simulink model "stm32_linker"  (R2025a)
settings: Solver=FixedStepAuto  StartTime=0.0  StopTime=inf  FixedStep=0.001  RelTol=1e-3
libraries: dspvision x3, instrumentseriallib x2, dspsnks4 x1, stmutilitieslib x1
settings Model: Creator=User  LastModifiedBy=User

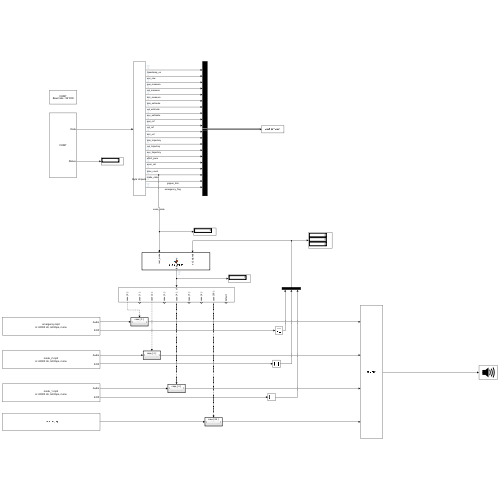
[thumbnail: Simulink's stored preview of the top-level diagram]
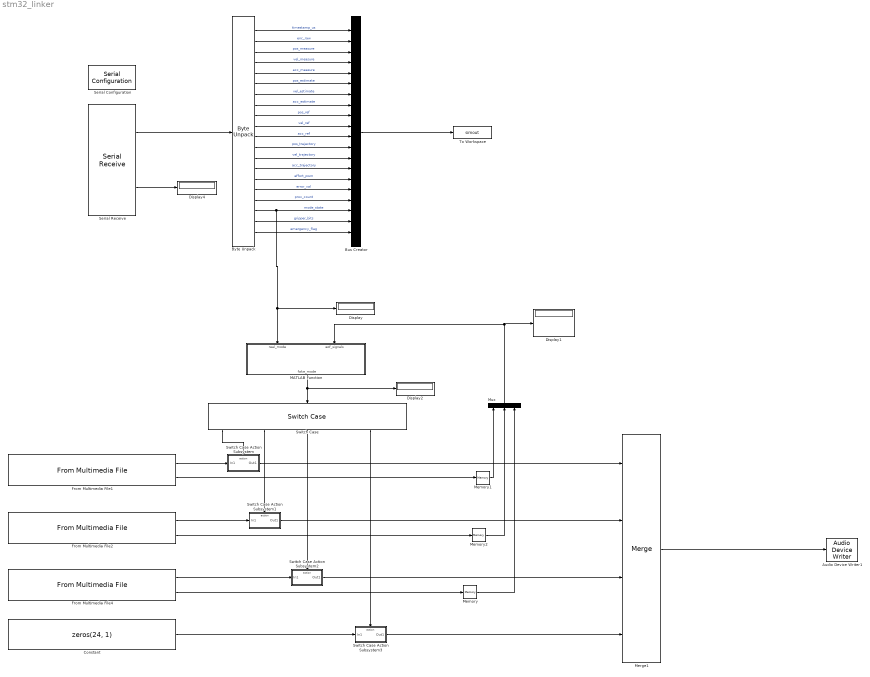
== system stm32_linker ==
  Audio Device Writer1 : dspsnks4/Audio Device Writer  Driver=DirectSound  Device=Headphones (Xiaomi Sound Party)  InheritSampleRate=on  SampleRate=44100  BitDepth=16-bit integer  BufferSize=4096  NumBuffers=10  DefaultOutputChannelMapping=on  OutputChannelMapping=1:2  OutputNumUnderrunSamples=off  DriverIdx=1  DeviceWarnFlag=''
  Bus Creator : BusCreator  Inputs=20
  Byte Unpack : stmutilitieslib/Byte Unpack  dimensions={1, 1, 1, 1, 1, 1, 1, 1, 1, 1, 1, 1, 1, 1, 1, 1, 1,1,1,1}  datatypes={'uint32', 'int32', 'single', 'single', 'single', 'single', 'single', 'single', 'single', 'single', 'single', 'single', 'single', 'single', 'single', 'single', 'int16', 'uint16', 'uint8', 'uint8'}  byteAlign=1  blockPlatform=stm32f4discovery
  Constant : Constant  Value=zeros(24, 1)
  Display{,1..2,4} (4 alike) : Display
  From Multimedia File1 : dspvision/From Multimedia File  inputFilename=C:\Users\User\Documents\GitHub\studioG4_system_modelling\MATLAB_DEBUGGER\mp3\emergency.mp3  readRange=[1 Inf]  loop=on  numPlays=inf  outputStreams=Audio only  videoDataType=single  audioDataType=double  inheritSampleTime=off  userDefinedSampleTime=0.001  noAudioOutput=off  isIntensityVideo=off  fourcc=RGB  colorVideoFormat=Separate color signals  outputEOF=on  dataOrg=Column-major  audioFrameSize=24  computeAudioFrameSize=off  outSamplingMode=Sample based
      settings: LibrarySourceBlock=audiosources/From Multimedia File
  From Multimedia File2 : dspvision/From Multimedia File  inputFilename=C:\Users\User\Documents\GitHub\studioG4_system_modelling\MATLAB_DEBUGGER\mp3\mode_2.mp3  readRange=[1 Inf]  loop=on  numPlays=inf  outputStreams=Audio only  videoDataType=single  audioDataType=double  inheritSampleTime=off  userDefinedSampleTime=0.001  noAudioOutput=off  isIntensityVideo=off  fourcc=RGB  colorVideoFormat=Separate color signals  outputEOF=on  dataOrg=Column-major  audioFrameSize=24  computeAudioFrameSize=off  outSamplingMode=Sample based
      settings: LibrarySourceBlock=audiosources/From Multimedia File
  From Multimedia File4 : dspvision/From Multimedia File  inputFilename=C:\Users\User\Documents\GitHub\studioG4_system_modelling\MATLAB_DEBUGGER\mp3\mode_1.mp3  readRange=[1 Inf]  loop=on  numPlays=inf  outputStreams=Audio only  videoDataType=single  audioDataType=double  inheritSampleTime=off  userDefinedSampleTime=0.001  noAudioOutput=off  isIntensityVideo=off  fourcc=RGB  colorVideoFormat=Separate color signals  outputEOF=on  dataOrg=Column-major  audioFrameSize=24  computeAudioFrameSize=off  outSamplingMode=Sample based
      settings: LibrarySourceBlock=audiosources/From Multimedia File
  MATLAB Function : MATLAB Function  TreatAsAtomicUnit=on
  Memory : Memory
  Memory1 : Memory
  Memory2 : Memory
  Merge1 : Merge  Inputs=4
  Mux : Mux  Inputs=3
  Serial Configuration : instrumentseriallib/Serial Configuration  Priority=-200000  PortSel=COM7  Port=COM7  ComPort=COM7  BaudRate=921000  DataBits=8  Parity=none  StopBits=1  ByteOrder=little-endian  FlowControl=none  Timeout=10  SimulateUsing=Interpreted execution  BlockInModel=on  aMode=1
      settings: LibrarySourceBlock=embeddedtargetslib/Host Communication/Serial Configuration
  Serial Receive : instrumentseriallib/Serial Receive  Priority=1  PortSel=COM7  Port=COM7  ComPort=COM7  DataType=uint8  SaveDataType=uint8  ToggleHeader=on  Header=[170 170 170 170]  ToggleDataSize=on  DataSize=[70 1]  ToggleTerminator=off  Terminator=Custom terminator  CustomTerminator=[]  InputFormat=Column major  EnableBlockingMode=off  ActionDataUnavailable=Output last received value  ActionWhenDataUnavailable=Output last received value  CustomValue=0  SampleTime=0.001  SimulateUsing=Interpreted execution  BlockInModel=on  aMode=1  LibraryInUse=instrumentlib
      settings: LibrarySourceBlock=embeddedtargetslib/Host Communication/Serial Receive
  Switch Case : SwitchCase  CaseConditions={0,1,2,3,4,5,6,99}
  Switch Case Action Subsystem : Subsystem  TreatAsAtomicUnit=on
  Switch Case Action Subsystem1 : Subsystem  TreatAsAtomicUnit=on
  Switch Case Action Subsystem2 : Subsystem  TreatAsAtomicUnit=on
  Switch Case Action Subsystem3 : Subsystem  TreatAsAtomicUnit=on
  To Workspace : ToWorkspace  VariableName=simout  SaveFormat=Timeseries  SampleTime=-1
  wires:
  Bus Creator/1 -> To Workspace/1
  Serial Receive/1 -> Byte Unpack/1
  Serial Receive/2 -> Display4/1
  Byte Unpack/1 -> Bus Creator/1  "timestamp_us"
  Byte Unpack/2 -> Bus Creator/2  "enc_raw"
  Byte Unpack/3 -> Bus Creator/3  "pos_measure"
  Byte Unpack/4 -> Bus Creator/4  "vel_measure"
  Byte Unpack/5 -> Bus Creator/5  "acc_measure"
  Byte Unpack/6 -> Bus Creator/6  "pos_estimate"
  Byte Unpack/7 -> Bus Creator/7  "vel_estimate"
  Byte Unpack/8 -> Bus Creator/8  "acc_estimate"
  Byte Unpack/9 -> Bus Creator/9  "pos_ref"
  Byte Unpack/10 -> Bus Creator/10  "vel_ref"
  Byte Unpack/11 -> Bus Creator/11  "acc_ref"
  Byte Unpack/12 -> Bus Creator/12  "pos_trajectory"
  Byte Unpack/13 -> Bus Creator/13  "vel_trajectory"
  Byte Unpack/14 -> Bus Creator/14  "acc_trajectory"
  Byte Unpack/15 -> Bus Creator/15  "effort_pwm"
  Byte Unpack/16 -> Bus Creator/16  "error_val"
  Byte Unpack/17 -> Bus Creator/17  "prox_count"
  Byte Unpack/18 -> Bus Creator/18, Display/1, MATLAB Function/1(real_mode)  "mode_state"
  Byte Unpack/19 -> Bus Creator/19  "gripper_bits"
  Byte Unpack/20 -> Bus Creator/20  "emergency_flag"
  Merge1/1 -> Audio Device Writer1/1
  From Multimedia File1/1 -> Switch Case Action Subsystem/1(In1)
  From Multimedia File2/1 -> Switch Case Action Subsystem1/1(In1)
  From Multimedia File4/1 -> Switch Case Action Subsystem2/1(In1)
  Switch Case Action Subsystem2/1(Out1) -> Merge1/3
  Switch Case Action Subsystem1/1(Out1) -> Merge1/2
  Switch Case Action Subsystem/1(Out1) -> Merge1/1
  Switch Case/3 -> Switch Case Action Subsystem1/Action
  From Multimedia File4/2 -> Memory/1
  From Multimedia File2/2 -> Memory2/1
  From Multimedia File1/2 -> Memory1/1
  Memory1/1 -> Mux/1
  Memory2/1 -> Mux/2
  Memory/1 -> Mux/3
  Mux/1 -> MATLAB Function/2(eof_signals), Display1/1
  MATLAB Function/1(fake_mode) -> Display2/1, Switch Case/1
  Switch Case/5 -> Switch Case Action Subsystem2/Action
  Switch Case/8 -> Switch Case Action Subsystem3/Action
  Switch Case Action Subsystem3/1(Out1) -> Merge1/4
  Constant/1 -> Switch Case Action Subsystem3/1(In1)
  Switch Case/1 -> Switch Case Action Subsystem/Action

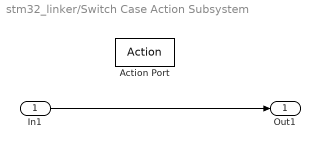
== system stm32_linker/Switch Case Action Subsystem ==
  In1 : Inport
  Action Port : ActionPort  InitializeStates=reset  ActionPortLabel=case [ 0 ]:
  Out1 : Outport
  wires:
  In1/1 -> Out1/1

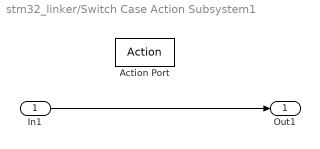
== system stm32_linker/Switch Case Action Subsystem1 ==
  In1 : Inport
  Action Port : ActionPort  InitializeStates=reset  ActionPortLabel=case [ 2 ]:
  Out1 : Outport
  wires:
  In1/1 -> Out1/1

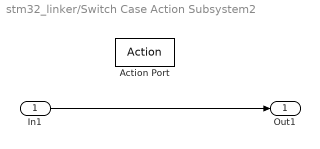
== system stm32_linker/Switch Case Action Subsystem2 ==
  In1 : Inport
  Action Port : ActionPort  InitializeStates=reset  ActionPortLabel=case [ 4 ]:
  Out1 : Outport
  wires:
  In1/1 -> Out1/1

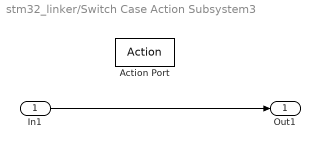
== system stm32_linker/Switch Case Action Subsystem3 ==
  In1 : Inport
  Action Port : ActionPort  InitializeStates=reset  ActionPortLabel=case [ 99 ]:
  Out1 : Outport
  wires:
  In1/1 -> Out1/1

== matlab function stm32_linker/MATLAB Function ==
  data: real_mode input; fake_mode output; eof_signals input
function fake_mode = audio_faker(real_mode, eof_signals)
    % persistent memory now tracks the count of plays
    persistent current_fake play_count last_real eof_latched;
    
    % Target: Play 2 times
    target_count = 2;
    
    if isempty(current_fake)
        current_fake = uint16(99); 
        play_count = zeros(1, 3);  % Tracks play count for 3 modes
        last_real = uint16(888);
        eof_latched = false(1, 3); % Prevents double-counting a single EOF pulse
    end

    % 1. RESET LOGIC
    % When the physical mode changes, reset the counter for that specific mode
    if real_mode ~= last_real
        last_real = real_mode;
        switch real_mode
            case 0, play_count(1) = 0;
            case 4, play_count(2) = 0;
            case 2, play_count(3) = 0;
        end
    end

    % 2. MAPPING
    idx = 0; 
    switch real_mode
        case 0, idx = 1;
        case 4, idx = 2;
        case 2, idx = 3;
    end

    % 3. COUNTER & SILENCING LOGIC
    if idx > 0 && idx <= length(eof_signals)
        
        % Detect EOF pulse and increment counter
        % eof_latched ensures we only count once per EOF trigger
        if eof_signals(idx) && ~eof_latched(idx)
            play_count(idx) = play_count(idx) + 1;
            eof_latched(idx) = true;
        elseif ~eof_signals(idx)
            % Clear latch when EOF signal returns to 0
            eof_latched(idx) = false;
        end

        % Decide output: Only switch to 99 if we hit the target
        if play_count(idx) >= target_count
            current_fake = uint16(99);
        else
            current_fake = uint16(real_mode);
        end
    else
        current_fake = uint16(99);
    end

    fake_mode = current_fake;
end
